simulink model "lecture05_9"  (R2020a)
settings: Solver=VariableStepAuto  StartTime=0.0  StopTime=10.0  MaxStep=1e-3  RelTol=1e-3
values from neighbouring files (symbols this model uses):
  Acl = A-B*K    [lecture05_11.m]    (also in lecture05_8.m)
  Bcl = B*K*Nx    [lecture05_11.m]    (also in lecture05_8.m)
  Ccl = C    [lecture05_11.m]    (also in lecture05_8.m)
  Dcl = D*K*Nx    [lecture05_11.m]    (also in lecture05_8.m)
  K = tf(numK, denK)    [lecture02_5.m]    (also in lecture05_1.m = Kp+Kd+Ki/s; lecture05_11.m = place(A,B,p); lecture05_2.m = Kp+Kd+Ki/s; lecture05_3.m = Kp+Kd+Ki/s)
settings Model: Creator=JY  LastModifiedBy=JY

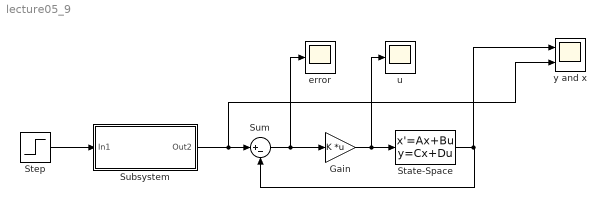
== system lecture05_9 ==
  Gain : Gain  Gain=K  Multiplication=Matrix(K*u)
  State-Space : StateSpace  A=Acl  B=Bcl  C=Ccl  D=Dcl  InitialCondition=0
  Step : Step  SampleTime=0
  Subsystem : Subsystem
  Sum : Sum  Inputs=|+-
  error : Scope
  u : Scope
  y and x : Scope  NumInputPorts=2
  wires:
  Sum/1 -> error/1, Gain/1
  Gain/1 -> u/1, State-Space/1
  State-Space/1 -> y and x/1, Sum/2
  Step/1 -> Subsystem/1(In1)
  Subsystem/1(Out2) -> y and x/2, Sum/1

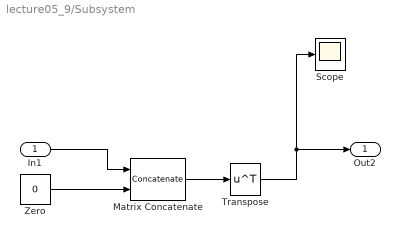
== system lecture05_9/Subsystem ==
  In1 : Inport
  Matrix Concatenate : Concatenate  Mode=Multidimensional array  ConcatenateDimension=2
  Scope : Scope
  Transpose : Math  Operator=transpose  SaturateOnIntegerOverflow=on
  Zero : Constant  Value=0  OutDataTypeStr=Inherit: Inherit via back propagation
  Out2 : Outport
  wires:
  In1/1 -> Matrix Concatenate/1
  Zero/1 -> Matrix Concatenate/2
  Matrix Concatenate/1 -> Transpose/1
  Transpose/1 -> Scope/1, Out2/1
